simulink model "Allocation_Test"  (R2015a)
settings: Solver=ode45  StartTime=0.0  StopTime=10.0  RelTol=1e-3
undefined symbols (not defined in the file or in its folder): magnitude
libraries: aerolibutil x10, simulink_extras x6, simulink x2
settings Model: Creator=Nick  LastModifiedBy=Nick

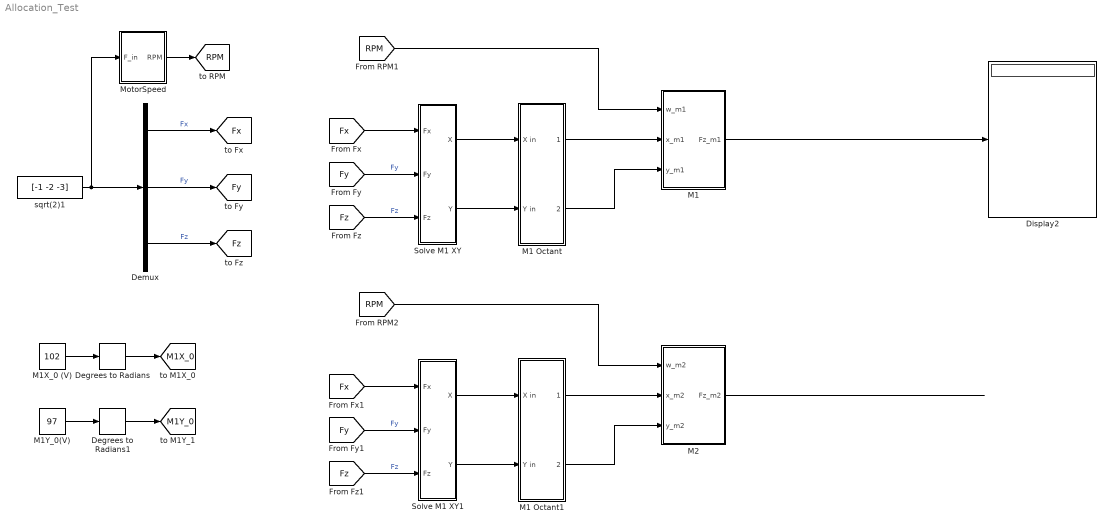
== system Allocation_Test ==
  Degrees to Radians : simulink_extras/Transformations/Degrees to Radians
  Degrees to Radians1 : simulink_extras/Transformations/Degrees to Radians
  Demux : Demux  Outputs=3
  Display2 : Display
      settings: Decimation=4
  M1 : Subsystem
  M1 Octant : Subsystem
  M1 Octant1 : Subsystem
  M1X_0 (V) : Constant  Value=102
  M1Y_0(V) : Constant  Value=97
  M2 : Subsystem
  MotorSpeed : Subsystem
  Solve M1 XY : Subsystem
  Solve M1 XY1 : Subsystem
  sqrt(2)1 : Constant  Value=[-1 -2 -3]
  tag scope: Fx=global, Fy=global, Fz=global, M1X_0=global, M1Y_0=global, RPM=global
  wires:
  sqrt(2)1/1 -> Demux/1, MotorSpeed/1(F_in)
  Demux/1 -> [Fx]  "Fx"
  Demux/2 -> [Fy]  "Fy"
  Demux/3 -> [Fz]  "Fz"
  MotorSpeed/1(RPM) -> [RPM]
  [Fz] -> Solve M1 XY/3(Fz)  "Fz"
  [Fx] -> Solve M1 XY/1(Fx)
  [Fy] -> Solve M1 XY/2(Fy)  "Fy"
  Solve M1 XY/2(Y) -> M1 Octant/2(Y in)
  Solve M1 XY/1(X) -> M1 Octant/1(X in)
  M1X_0 (V)/1 -> Degrees to Radians/1
  Degrees to Radians/1 -> [M1X_0]
  M1Y_0(V)/1 -> Degrees to Radians1/1
  Degrees to Radians1/1 -> [M1Y_0]
  [RPM] -> M1/1(w_m1)
  M1 Octant/2(Y Out) -> M1/3(y_m1)
  M1 Octant/1(X Out) -> M1/2(x_m1)
  M1/1(Fz_m1) -> Display2/1
  [Fz] -> Solve M1 XY1/3(Fz)  "Fz"
  [Fx] -> Solve M1 XY1/1(Fx)
  [Fy] -> Solve M1 XY1/2(Fy)  "Fy"
  Solve M1 XY1/2(Y) -> M1 Octant1/2(Y in)
  Solve M1 XY1/1(X) -> M1 Octant1/1(X in)
  [RPM] -> M2/1(w_m2)
  M1 Octant1/2(Y Out) -> M2/3(y_m2)
  M1 Octant1/1(X Out) -> M2/2(x_m2)
  M2/1(Fz_m2) -> ?

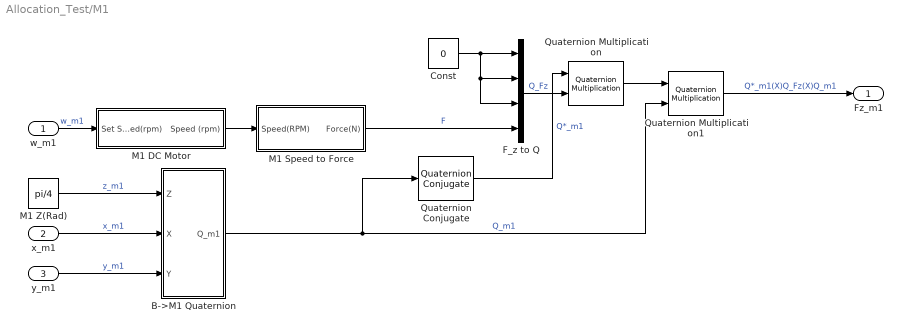
== system Allocation_Test/M1 ==
  w_m1 : Inport
  x_m1 : Inport  Port=2
  y_m1 : Inport  Port=3
  B->M1 Quaternion : Subsystem
  Const : Constant  Value=0
  F_z to Q : Concatenate  NumInputs=4
  M1 DC Motor : Subsystem
  M1 Speed to Force : Subsystem
  M1 Z(Rad) : Constant  Value=pi/4
  Quaternion Conjugate : aerolibutil/Quaternion Conjugate
  Quaternion Multiplication : aerolibutil/Quaternion Multiplication
  Quaternion Multiplication1 : aerolibutil/Quaternion Multiplication
  Fz_m1 : Outport
  wires:
  Quaternion Multiplication/1 -> Quaternion Multiplication1/1
  Const/1 -> F_z to Q/1, F_z to Q/3, F_z to Q/2
  M1 DC Motor/1(Speed (rpm)) -> M1 Speed to Force/1(Speed(RPM))
  B->M1 Quaternion/1(Q_m1) -> Quaternion Multiplication1/2, Quaternion Conjugate/1  "Q_m1"
  w_m1/1 -> M1 DC Motor/1(Set Speed(rpm))  "w_m1"
  F_z to Q/1 -> Quaternion Multiplication/2  "Q_Fz"
  M1 Z(Rad)/1 -> B->M1 Quaternion/1("Z ")  "z_m1"
  M1 Speed to Force/1(Force(N)) -> F_z to Q/4  "F"
  y_m1/1 -> B->M1 Quaternion/3(Y)  "y_m1"
  Quaternion Multiplication1/1 -> Fz_m1/1  "Q*_m1(X)Q_Fz(X)Q_m1"
  x_m1/1 -> B->M1 Quaternion/2(X)  "x_m1"
  Quaternion Conjugate/1 -> Quaternion Multiplication/1  "Q*_m1"

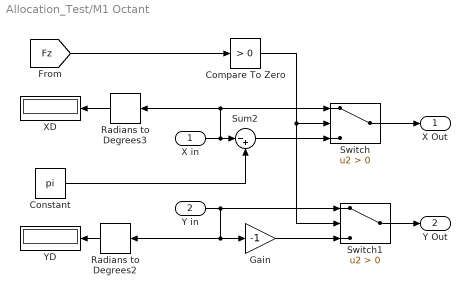
== system Allocation_Test/M1 Octant ==
  X in : Inport
  Y in : Inport  Port=2
  Compare To Zero : simulink/Logic and Bit Operations/Compare To Zero  relop=>  OutDataTypeStr=boolean
  Constant : Constant  Value=pi
  Gain : Gain  Gain=-1
  Radians to Degrees2 : simulink_extras/Transformations/Radians to Degrees
  Radians to Degrees3 : simulink_extras/Transformations/Radians to Degrees
  Sum2 : Sum  Inputs=|-+
  Switch : Switch  Criteria=u2 > Threshold
  Switch1 : Switch  Criteria=u2 > Threshold
  XD : Display
  YD : Display
  X Out : Outport
  Y Out : Outport  Port=2
  wires:
  Radians to Degrees2/1 -> YD/1
  Radians to Degrees3/1 -> XD/1
  Switch1/1 -> Y Out/1
  Sum2/1 -> Switch/3
  X in/1 -> Sum2/1, Switch/1, Radians to Degrees3/1
  Y in/1 -> Radians to Degrees2/1, Gain/1, Switch1/1
  Constant/1 -> Sum2/2
  Switch/1 -> X Out/1
  Gain/1 -> Switch1/3
  Compare To Zero/1 -> Switch1/2, Switch/2
  [Fz] -> Compare To Zero/1

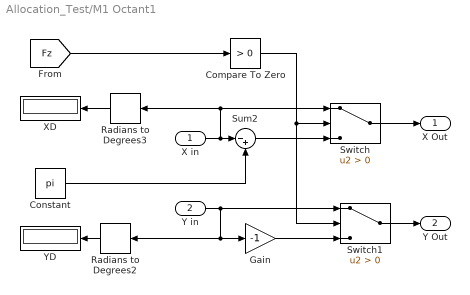
== system Allocation_Test/M1 Octant1 ==
  X in : Inport
  Y in : Inport  Port=2
  Compare To Zero : simulink/Logic and Bit Operations/Compare To Zero  relop=>  OutDataTypeStr=boolean
  Constant : Constant  Value=pi
  Gain : Gain  Gain=-1
  Radians to Degrees2 : simulink_extras/Transformations/Radians to Degrees
  Radians to Degrees3 : simulink_extras/Transformations/Radians to Degrees
  Sum2 : Sum  Inputs=|-+
  Switch : Switch  Criteria=u2 > Threshold
  Switch1 : Switch  Criteria=u2 > Threshold
  XD : Display
  YD : Display
  X Out : Outport
  Y Out : Outport  Port=2
  wires:
  Radians to Degrees2/1 -> YD/1
  Radians to Degrees3/1 -> XD/1
  Switch1/1 -> Y Out/1
  Sum2/1 -> Switch/3
  X in/1 -> Sum2/1, Switch/1, Radians to Degrees3/1
  Y in/1 -> Radians to Degrees2/1, Gain/1, Switch1/1
  Constant/1 -> Sum2/2
  Switch/1 -> X Out/1
  Gain/1 -> Switch1/3
  Compare To Zero/1 -> Switch1/2, Switch/2
  [Fz] -> Compare To Zero/1

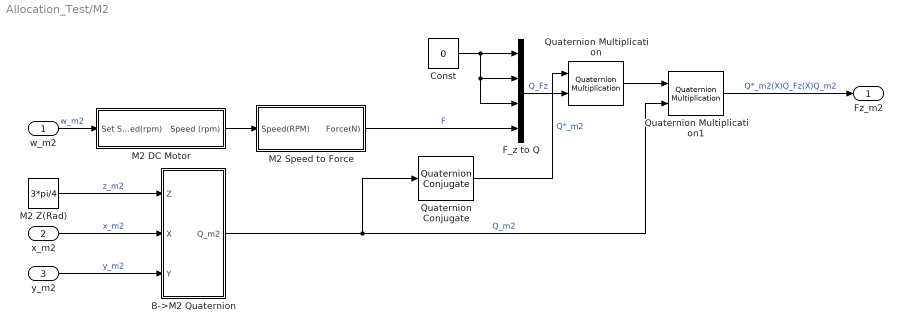
== system Allocation_Test/M2 ==
  w_m2 : Inport
  x_m2 : Inport  Port=2
  y_m2 : Inport  Port=3
  B->M2 Quaternion : Subsystem
  Const : Constant  Value=0
  F_z to Q : Concatenate  NumInputs=4
  M2 DC Motor : Subsystem
  M2 Speed to Force : Subsystem
  M2 Z(Rad) : Constant  Value=3*pi/4
  Quaternion Conjugate : aerolibutil/Quaternion Conjugate
  Quaternion Multiplication : aerolibutil/Quaternion Multiplication
  Quaternion Multiplication1 : aerolibutil/Quaternion Multiplication
  Fz_m2 : Outport
  wires:
  Quaternion Multiplication/1 -> Quaternion Multiplication1/1
  Const/1 -> F_z to Q/1, F_z to Q/3, F_z to Q/2
  M2 DC Motor/1(Speed (rpm)) -> M2 Speed to Force/1(Speed(RPM))
  B->M2 Quaternion/1(Q_m2) -> Quaternion Multiplication1/2, Quaternion Conjugate/1  "Q_m2"
  w_m2/1 -> M2 DC Motor/1(Set Speed(rpm))  "w_m2"
  F_z to Q/1 -> Quaternion Multiplication/2  "Q_Fz"
  M2 Z(Rad)/1 -> B->M2 Quaternion/1("Z ")  "z_m2"
  M2 Speed to Force/1(Force(N)) -> F_z to Q/4  "F"
  y_m2/1 -> B->M2 Quaternion/3(Y)  "y_m2"
  Quaternion Multiplication1/1 -> Fz_m2/1  "Q*_m2(X)Q_Fz(X)Q_m2"
  x_m2/1 -> B->M2 Quaternion/2(X)  "x_m2"
  Quaternion Conjugate/1 -> Quaternion Multiplication/1  "Q*_m2"

== system Allocation_Test/MotorSpeed ==
  F_in : Inport
  Divide : Product  Inputs=*/
  Force Coefficient CT : Constant  Value=0.000243
  Mins : Constant  Value=60
  Product : Product
  w^2 : Sqrt  SaturateOnIntegerOverflow=on
  |F| : Sqrt  SaturateOnIntegerOverflow=on
  |F|^2 : DotProduct  InputSameDT=on  OutDataTypeStr=Inherit: Inherit via internal rule
  RPM : Outport
  wires:
  w^2/1 -> Product/2
  Product/1 -> RPM/1  "RPM"
  Mins/1 -> Product/1
  Divide/1 -> w^2/1
  Force Coefficient CT/1 -> Divide/2
  F_in/1 -> |F|^2/2, |F|^2/1
  |F|^2/1 -> |F|/1
  |F|/1 -> Divide/1

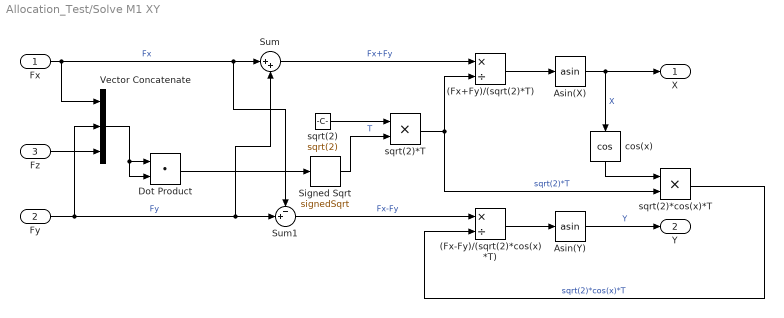
== system Allocation_Test/Solve M1 XY ==
  Fx : Inport
  Fy : Inport  Port=2
  Fz : Inport  Port=3
  (Fx+Fy)/(sqrt(2)*T) : Product  Inputs=*/
  (Fx-Fy)/(sqrt(2)*cos(x)*T) : Product  Inputs=*/
  Asin(X) : Trigonometry  Operator=asin
  Asin(Y) : Trigonometry  Operator=asin
  Dot Product : DotProduct  InputSameDT=on  OutDataTypeStr=Inherit: Inherit via internal rule
  Signed Sqrt : Sqrt  Operator=signedSqrt  SaturateOnIntegerOverflow=on
  Sum : Sum  Inputs=|++
  Sum1 : Sum  Inputs=-+|
  Vector Concatenate : Concatenate  NumInputs=3
  cos(x) : Trigonometry  Operator=cos
  sqrt(2) : Constant  Value=sqrt(2)
  sqrt(2)*T : Product
  sqrt(2)*cos(x)*T : Product
  X : Outport
  Y : Outport  Port=2
  wires:
  Fy/1 -> Vector Concatenate/2, Sum/2, Sum1/2  "Fy"
  Sum/1 -> (Fx+Fy)/(sqrt(2)*T)/1  "Fx+Fy"
  sqrt(2)/1 -> sqrt(2)*T/1
  cos(x)/1 -> sqrt(2)*cos(x)*T/1
  sqrt(2)*T/1 -> (Fx+Fy)/(sqrt(2)*T)/2, sqrt(2)*cos(x)*T/2  "sqrt(2)*T"
  (Fx+Fy)/(sqrt(2)*T)/1 -> Asin(X)/1
  sqrt(2)*cos(x)*T/1 -> (Fx-Fy)/(sqrt(2)*cos(x)*T)/2  "sqrt(2)*cos(x)*T"
  (Fx-Fy)/(sqrt(2)*cos(x)*T)/1 -> Asin(Y)/1
  Sum1/1 -> (Fx-Fy)/(sqrt(2)*cos(x)*T)/1  "Fx-Fy"
  Asin(Y)/1 -> Y/1  "Y"
  Asin(X)/1 -> X/1, cos(x)/1  "X"
  Fz/1 -> Vector Concatenate/3
  Signed Sqrt/1 -> sqrt(2)*T/2  "T"
  Fx/1 -> Sum1/1, Sum/1, Vector Concatenate/1  "Fx"
  Vector Concatenate/1 -> Dot Product/2, Dot Product/1
  Dot Product/1 -> Signed Sqrt/1

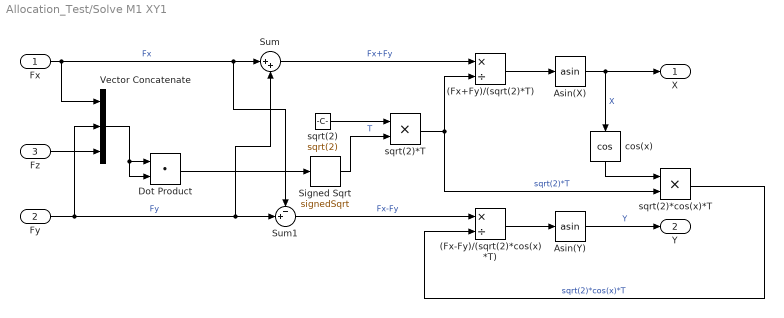
== system Allocation_Test/Solve M1 XY1 ==
  Fx : Inport
  Fy : Inport  Port=2
  Fz : Inport  Port=3
  (Fx+Fy)/(sqrt(2)*T) : Product  Inputs=*/
  (Fx-Fy)/(sqrt(2)*cos(x)*T) : Product  Inputs=*/
  Asin(X) : Trigonometry  Operator=asin
  Asin(Y) : Trigonometry  Operator=asin
  Dot Product : DotProduct  InputSameDT=on  OutDataTypeStr=Inherit: Inherit via internal rule
  Signed Sqrt : Sqrt  Operator=signedSqrt  SaturateOnIntegerOverflow=on
  Sum : Sum  Inputs=|++
  Sum1 : Sum  Inputs=-+|
  Vector Concatenate : Concatenate  NumInputs=3
  cos(x) : Trigonometry  Operator=cos
  sqrt(2) : Constant  Value=sqrt(2)
  sqrt(2)*T : Product
  sqrt(2)*cos(x)*T : Product
  X : Outport
  Y : Outport  Port=2
  wires:
  Fy/1 -> Vector Concatenate/2, Sum/2, Sum1/2  "Fy"
  Sum/1 -> (Fx+Fy)/(sqrt(2)*T)/1  "Fx+Fy"
  sqrt(2)/1 -> sqrt(2)*T/1
  cos(x)/1 -> sqrt(2)*cos(x)*T/1
  sqrt(2)*T/1 -> (Fx+Fy)/(sqrt(2)*T)/2, sqrt(2)*cos(x)*T/2  "sqrt(2)*T"
  (Fx+Fy)/(sqrt(2)*T)/1 -> Asin(X)/1
  sqrt(2)*cos(x)*T/1 -> (Fx-Fy)/(sqrt(2)*cos(x)*T)/2  "sqrt(2)*cos(x)*T"
  (Fx-Fy)/(sqrt(2)*cos(x)*T)/1 -> Asin(Y)/1
  Sum1/1 -> (Fx-Fy)/(sqrt(2)*cos(x)*T)/1  "Fx-Fy"
  Asin(Y)/1 -> Y/1  "Y"
  Asin(X)/1 -> X/1, cos(x)/1  "X"
  Fz/1 -> Vector Concatenate/3
  Signed Sqrt/1 -> sqrt(2)*T/2  "T"
  Fx/1 -> Sum1/1, Sum/1, Vector Concatenate/1  "Fx"
  Vector Concatenate/1 -> Dot Product/2, Dot Product/1
  Dot Product/1 -> Signed Sqrt/1

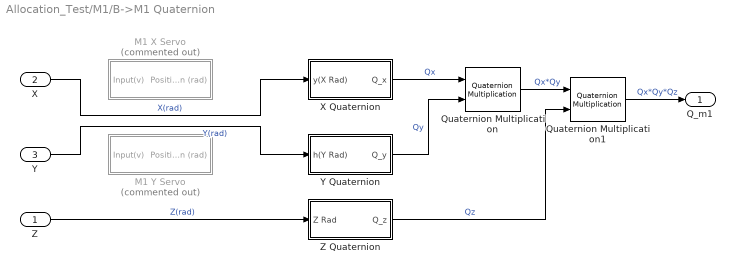
== system Allocation_Test/M1/B->M1 Quaternion ==
  "Z " : Inport
  X : Inport  Port=2
  Y : Inport  Port=3
  "M1 X Servo " : Subsystem  Commented=on
  M1 Y Servo : Subsystem  Commented=on
  Quaternion Multiplication : aerolibutil/Quaternion Multiplication
  Quaternion Multiplication1 : aerolibutil/Quaternion Multiplication
  X Quaternion : Subsystem
  Y Quaternion : Subsystem
  Z Quaternion : Subsystem
  Q_m1 : Outport
  wires:
  X/1 -> X Quaternion/1(y(X Rad))  "X(rad)"
  "Z "/1 -> Z Quaternion/1(Z Rad)  "Z(rad)"
  Quaternion Multiplication/1 -> Quaternion Multiplication1/1  "Qx*Qy"
  Quaternion Multiplication1/1 -> Q_m1/1  "Qx*Qy*Qz"
  Y/1 -> Y Quaternion/1(h(Y Rad))  "Y(rad)"
  X Quaternion/1(Q_x) -> Quaternion Multiplication/1  "Qx"
  Y Quaternion/1(Q_y) -> Quaternion Multiplication/2  "Qy"
  Z Quaternion/1(Q_z) -> Quaternion Multiplication1/2  "Qz"

== system Allocation_Test/M1/M1 DC Motor ==
  note: M1 DC Motor response
  Set Speed(rpm) : Inport
  ->ms : Product  Inputs=*/
  10080 Max : Saturate  UpperLimit=10080  LowerLimit=-10080
  Add : Sum
  Dead Time (ms) : Constant
  Dead Time Block : VariableTransportDelay  MaximumDelay=10
  Miliseconds : Constant  Value=1000
  Starting Speed : Constant  Value=10080
  Subtract : Sum  Inputs=+-
  Transfer Fcn : TransferFcn  Numerator=1  Denominator=[0.6 1]
  Speed (rpm) : Outport
  wires:
  Dead Time Block/1 -> Transfer Fcn/1
  Miliseconds/1 -> ->ms/2
  Dead Time (ms)/1 -> ->ms/1
  ->ms/1 -> Dead Time Block/2
  Transfer Fcn/1 -> 10080 Max/1
  Set Speed(rpm)/1 -> Subtract/1
  10080 Max/1 -> Add/1
  Add/1 -> Speed (rpm)/1
  Starting Speed/1 -> Add/2, Subtract/2
  Subtract/1 -> Dead Time Block/1

== system Allocation_Test/M1/M1 Speed to Force ==
  note: RPS to Force
  Speed(RPM) : Inport
  ->RPS : Product  Inputs=*/
  Force Coefficient CT : Constant  Value=0.000243
  M1 w^2 : Math  Operator=magnitude^2  SaturateOnIntegerOverflow=on
  Mins : Constant  Value=60
  Product : Product
  Force(N) : Outport
  wires:
  M1 w^2/1 -> Product/2
  ->RPS/1 -> M1 w^2/1
  Speed(RPM)/1 -> ->RPS/1
  Force Coefficient CT/1 -> Product/1
  Mins/1 -> ->RPS/2
  Product/1 -> Force(N)/1

== system Allocation_Test/M2/B->M2 Quaternion ==
  "Z " : Inport
  X : Inport  Port=2
  Y : Inport  Port=3
  "M1 X Servo " : Subsystem  Commented=on
  M1 Y Servo : Subsystem  Commented=on
  Quaternion Multiplication : aerolibutil/Quaternion Multiplication
  Quaternion Multiplication1 : aerolibutil/Quaternion Multiplication
  X Quaternion : Subsystem
  Y Quaternion : Subsystem
  Z Quaternion : Subsystem
  Q_m2 : Outport
  wires:
  X/1 -> X Quaternion/1(y(X Rad))  "X(rad)"
  "Z "/1 -> Z Quaternion/1(Z Rad)  "Z(rad)"
  Quaternion Multiplication/1 -> Quaternion Multiplication1/1  "Qx*Qy"
  Quaternion Multiplication1/1 -> Q_m2/1  "Qx*Qy*Qz"
  Y/1 -> Y Quaternion/1(h(Y Rad))  "Y(rad)"
  X Quaternion/1(Q_x) -> Quaternion Multiplication/1  "Qx"
  Y Quaternion/1(Q_y) -> Quaternion Multiplication/2  "Qy"
  Z Quaternion/1(Q_z) -> Quaternion Multiplication1/2  "Qz"

== system Allocation_Test/M2/M2 DC Motor ==
  note: M1 DC Motor response
  Set Speed(rpm) : Inport
  ->ms : Product  Inputs=*/
  10080 Max : Saturate  UpperLimit=10080  LowerLimit=-10080
  Add : Sum
  Dead Time (ms) : Constant
  Dead Time Block : VariableTransportDelay  MaximumDelay=10
  Miliseconds : Constant  Value=1000
  Starting Speed : Constant  Value=10080
  Subtract : Sum  Inputs=+-
  Transfer Fcn : TransferFcn  Numerator=1  Denominator=[0.6 1]
  Speed (rpm) : Outport
  wires:
  Dead Time Block/1 -> Transfer Fcn/1
  Miliseconds/1 -> ->ms/2
  Dead Time (ms)/1 -> ->ms/1
  ->ms/1 -> Dead Time Block/2
  Transfer Fcn/1 -> 10080 Max/1
  Set Speed(rpm)/1 -> Subtract/1
  10080 Max/1 -> Add/1
  Add/1 -> Speed (rpm)/1
  Starting Speed/1 -> Add/2, Subtract/2
  Subtract/1 -> Dead Time Block/1

== system Allocation_Test/M2/M2 Speed to Force ==
  note: RPS to Force
  Speed(RPM) : Inport
  ->RPS : Product  Inputs=*/
  Force Coefficient CT : Constant  Value=0.000243
  M1 w^2 : Math  Operator=magnitude^2  SaturateOnIntegerOverflow=on
  Mins : Constant  Value=60
  Product : Product
  Force(N) : Outport
  wires:
  M1 w^2/1 -> Product/2
  ->RPS/1 -> M1 w^2/1
  Speed(RPM)/1 -> ->RPS/1
  Force Coefficient CT/1 -> Product/1
  Mins/1 -> ->RPS/2
  Product/1 -> Force(N)/1

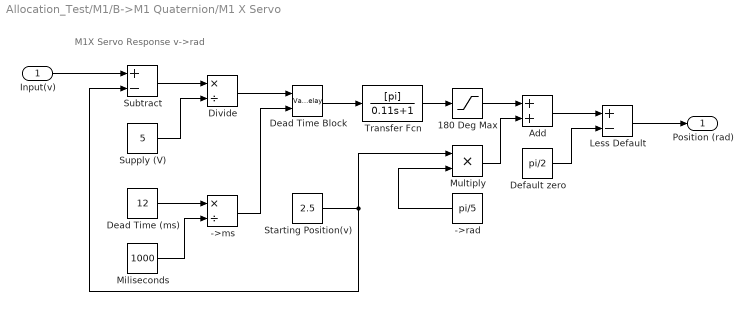
== system Allocation_Test/M1/B->M1 Quaternion/M1 X Servo  ==
  note: M1X Servo Response v->rad
  Input(v) : Inport
  ->ms : Product  Inputs=*/
  ->rad : Constant  Value=pi/5
  180 Deg Max : Saturate  UpperLimit=pi  LowerLimit=-pi
  Add : Sum
  Dead Time (ms) : Constant  Value=12
  Dead Time Block : VariableTransportDelay  MaximumDelay=10
  Default zero : Constant  Value=pi/2
  Divide : Product  Inputs=*/
  Less Default : Sum  Inputs=+-
  Miliseconds : Constant  Value=1000
  Multiply : Product  Inputs=**
  Starting Position(v) : Constant  Value=2.5
  Subtract : Sum  Inputs=+-
  Supply (V) : Constant  Value=5
  Transfer Fcn : TransferFcn  Numerator=[pi]  Denominator=[0.11 1]
  Position (rad) : Outport
  wires:
  Miliseconds/1 -> ->ms/2
  Dead Time (ms)/1 -> ->ms/1
  Default zero/1 -> Less Default/2
  Starting Position(v)/1 -> Multiply/1, Subtract/2
  Subtract/1 -> Divide/1
  Supply (V)/1 -> Divide/2
  Divide/1 -> Dead Time Block/1
  ->ms/1 -> Dead Time Block/2
  Dead Time Block/1 -> Transfer Fcn/1
  Transfer Fcn/1 -> 180 Deg Max/1
  180 Deg Max/1 -> Add/1
  ->rad/1 -> Multiply/2
  Multiply/1 -> Add/2
  Less Default/1 -> Position (rad)/1
  Add/1 -> Less Default/1
  Input(v)/1 -> Subtract/1

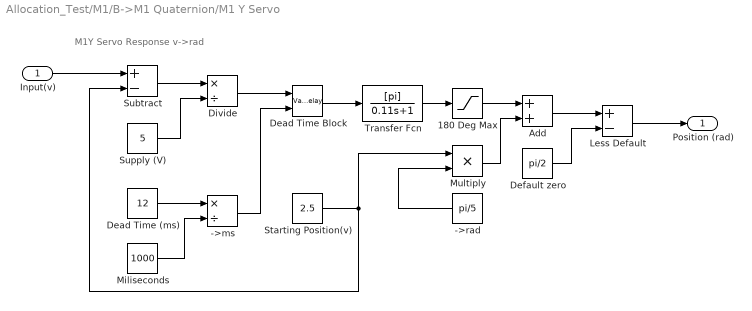
== system Allocation_Test/M1/B->M1 Quaternion/M1 Y Servo ==
  note: M1Y Servo Response v->rad
  Input(v) : Inport
  ->ms : Product  Inputs=*/
  ->rad : Constant  Value=pi/5
  180 Deg Max : Saturate  UpperLimit=pi  LowerLimit=-pi
  Add : Sum
  Dead Time (ms) : Constant  Value=12
  Dead Time Block : VariableTransportDelay  MaximumDelay=10
  Default zero : Constant  Value=pi/2
  Divide : Product  Inputs=*/
  Less Default : Sum  Inputs=+-
  Miliseconds : Constant  Value=1000
  Multiply : Product  Inputs=**
  Starting Position(v) : Constant  Value=2.5
  Subtract : Sum  Inputs=+-
  Supply (V) : Constant  Value=5
  Transfer Fcn : TransferFcn  Numerator=[pi]  Denominator=[0.11 1]
  Position (rad) : Outport
  wires:
  Miliseconds/1 -> ->ms/2
  Dead Time (ms)/1 -> ->ms/1
  Default zero/1 -> Less Default/2
  Starting Position(v)/1 -> Multiply/1, Subtract/2
  Subtract/1 -> Divide/1
  Supply (V)/1 -> Divide/2
  Divide/1 -> Dead Time Block/1
  ->ms/1 -> Dead Time Block/2
  Dead Time Block/1 -> Transfer Fcn/1
  Transfer Fcn/1 -> 180 Deg Max/1
  180 Deg Max/1 -> Add/1
  ->rad/1 -> Multiply/2
  Multiply/1 -> Add/2
  Less Default/1 -> Position (rad)/1
  Add/1 -> Less Default/1
  Input(v)/1 -> Subtract/1

== system Allocation_Test/M1/B->M1 Quaternion/X Quaternion ==
  y(X Rad) : Inport
  Const : Constant  Value=2
  Const1 : Constant  Value=0
  Divide : Product  Inputs=*/
  Trigonometric Function : Trigonometry  Operator=cos
  Trigonometric Function1 : Trigonometry
  Vector Concatenate : Concatenate  NumInputs=4
  Q_x : Outport
  wires:
  Vector Concatenate/1 -> Q_x/1
  Const/1 -> Divide/2
  Trigonometric Function1/1 -> Vector Concatenate/2
  Trigonometric Function/1 -> Vector Concatenate/1
  Const1/1 -> Vector Concatenate/4, Vector Concatenate/3
  Divide/1 -> Trigonometric Function1/1, Trigonometric Function/1
  y(X Rad)/1 -> Divide/1

== system Allocation_Test/M1/B->M1 Quaternion/Y Quaternion ==
  h(Y Rad) : Inport
  Const : Constant  Value=2
  Const1 : Constant  Value=0
  Divide : Product  Inputs=*/
  Trigonometric Function : Trigonometry  Operator=cos
  Trigonometric Function1 : Trigonometry
  Vector Concatenate : Concatenate  NumInputs=4
  Q_y : Outport
  wires:
  Vector Concatenate/1 -> Q_y/1
  Const/1 -> Divide/2
  Trigonometric Function/1 -> Vector Concatenate/1
  Const1/1 -> Vector Concatenate/2, Vector Concatenate/4
  Divide/1 -> Trigonometric Function1/1, Trigonometric Function/1
  h(Y Rad)/1 -> Divide/1
  Trigonometric Function1/1 -> Vector Concatenate/3

== system Allocation_Test/M1/B->M1 Quaternion/Z Quaternion ==
  Z Rad : Inport
  Const : Constant  Value=2
  Const1 : Constant  Value=0
  Divide : Product  Inputs=*/
  Trigonometric Function : Trigonometry  Operator=cos
  Trigonometric Function1 : Trigonometry
  Vector Concatenate : Concatenate  NumInputs=4
  Q_z : Outport
  wires:
  Vector Concatenate/1 -> Q_z/1
  Const/1 -> Divide/2
  Trigonometric Function/1 -> Vector Concatenate/1
  Const1/1 -> Vector Concatenate/3, Vector Concatenate/2
  Divide/1 -> Trigonometric Function1/1, Trigonometric Function/1
  Z Rad/1 -> Divide/1
  Trigonometric Function1/1 -> Vector Concatenate/4

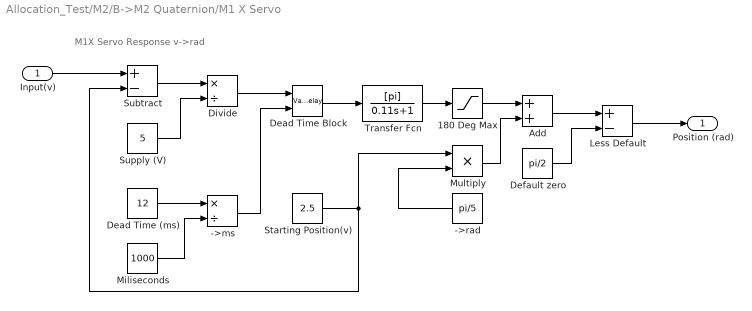
== system Allocation_Test/M2/B->M2 Quaternion/M1 X Servo  ==
  note: M1X Servo Response v->rad
  Input(v) : Inport
  ->ms : Product  Inputs=*/
  ->rad : Constant  Value=pi/5
  180 Deg Max : Saturate  UpperLimit=pi  LowerLimit=-pi
  Add : Sum
  Dead Time (ms) : Constant  Value=12
  Dead Time Block : VariableTransportDelay  MaximumDelay=10
  Default zero : Constant  Value=pi/2
  Divide : Product  Inputs=*/
  Less Default : Sum  Inputs=+-
  Miliseconds : Constant  Value=1000
  Multiply : Product  Inputs=**
  Starting Position(v) : Constant  Value=2.5
  Subtract : Sum  Inputs=+-
  Supply (V) : Constant  Value=5
  Transfer Fcn : TransferFcn  Numerator=[pi]  Denominator=[0.11 1]
  Position (rad) : Outport
  wires:
  Miliseconds/1 -> ->ms/2
  Dead Time (ms)/1 -> ->ms/1
  Default zero/1 -> Less Default/2
  Starting Position(v)/1 -> Multiply/1, Subtract/2
  Subtract/1 -> Divide/1
  Supply (V)/1 -> Divide/2
  Divide/1 -> Dead Time Block/1
  ->ms/1 -> Dead Time Block/2
  Dead Time Block/1 -> Transfer Fcn/1
  Transfer Fcn/1 -> 180 Deg Max/1
  180 Deg Max/1 -> Add/1
  ->rad/1 -> Multiply/2
  Multiply/1 -> Add/2
  Less Default/1 -> Position (rad)/1
  Add/1 -> Less Default/1
  Input(v)/1 -> Subtract/1

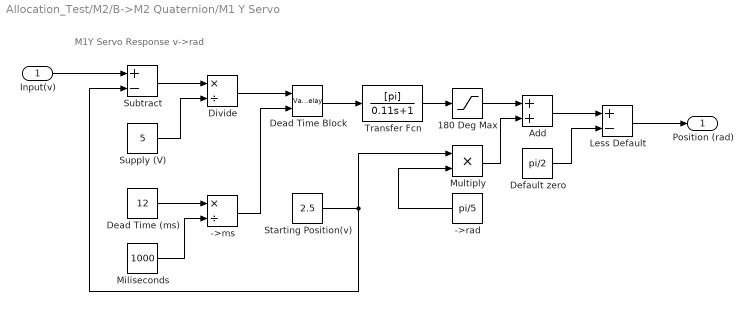
== system Allocation_Test/M2/B->M2 Quaternion/M1 Y Servo ==
  note: M1Y Servo Response v->rad
  Input(v) : Inport
  ->ms : Product  Inputs=*/
  ->rad : Constant  Value=pi/5
  180 Deg Max : Saturate  UpperLimit=pi  LowerLimit=-pi
  Add : Sum
  Dead Time (ms) : Constant  Value=12
  Dead Time Block : VariableTransportDelay  MaximumDelay=10
  Default zero : Constant  Value=pi/2
  Divide : Product  Inputs=*/
  Less Default : Sum  Inputs=+-
  Miliseconds : Constant  Value=1000
  Multiply : Product  Inputs=**
  Starting Position(v) : Constant  Value=2.5
  Subtract : Sum  Inputs=+-
  Supply (V) : Constant  Value=5
  Transfer Fcn : TransferFcn  Numerator=[pi]  Denominator=[0.11 1]
  Position (rad) : Outport
  wires:
  Miliseconds/1 -> ->ms/2
  Dead Time (ms)/1 -> ->ms/1
  Default zero/1 -> Less Default/2
  Starting Position(v)/1 -> Multiply/1, Subtract/2
  Subtract/1 -> Divide/1
  Supply (V)/1 -> Divide/2
  Divide/1 -> Dead Time Block/1
  ->ms/1 -> Dead Time Block/2
  Dead Time Block/1 -> Transfer Fcn/1
  Transfer Fcn/1 -> 180 Deg Max/1
  180 Deg Max/1 -> Add/1
  ->rad/1 -> Multiply/2
  Multiply/1 -> Add/2
  Less Default/1 -> Position (rad)/1
  Add/1 -> Less Default/1
  Input(v)/1 -> Subtract/1

== system Allocation_Test/M2/B->M2 Quaternion/X Quaternion ==
  y(X Rad) : Inport
  Const : Constant  Value=2
  Const1 : Constant  Value=0
  Divide : Product  Inputs=*/
  Trigonometric Function : Trigonometry  Operator=cos
  Trigonometric Function1 : Trigonometry
  Vector Concatenate : Concatenate  NumInputs=4
  Q_x : Outport
  wires:
  Vector Concatenate/1 -> Q_x/1
  Const/1 -> Divide/2
  Trigonometric Function1/1 -> Vector Concatenate/2
  Trigonometric Function/1 -> Vector Concatenate/1
  Const1/1 -> Vector Concatenate/4, Vector Concatenate/3
  Divide/1 -> Trigonometric Function1/1, Trigonometric Function/1
  y(X Rad)/1 -> Divide/1

== system Allocation_Test/M2/B->M2 Quaternion/Y Quaternion ==
  h(Y Rad) : Inport
  Const : Constant  Value=2
  Const1 : Constant  Value=0
  Divide : Product  Inputs=*/
  Trigonometric Function : Trigonometry  Operator=cos
  Trigonometric Function1 : Trigonometry
  Vector Concatenate : Concatenate  NumInputs=4
  Q_y : Outport
  wires:
  Vector Concatenate/1 -> Q_y/1
  Const/1 -> Divide/2
  Trigonometric Function/1 -> Vector Concatenate/1
  Const1/1 -> Vector Concatenate/2, Vector Concatenate/4
  Divide/1 -> Trigonometric Function1/1, Trigonometric Function/1
  h(Y Rad)/1 -> Divide/1
  Trigonometric Function1/1 -> Vector Concatenate/3

== system Allocation_Test/M2/B->M2 Quaternion/Z Quaternion ==
  Z Rad : Inport
  Const : Constant  Value=2
  Const1 : Constant  Value=0
  Divide : Product  Inputs=*/
  Trigonometric Function : Trigonometry  Operator=cos
  Trigonometric Function1 : Trigonometry
  Vector Concatenate : Concatenate  NumInputs=4
  Q_z : Outport
  wires:
  Vector Concatenate/1 -> Q_z/1
  Const/1 -> Divide/2
  Trigonometric Function/1 -> Vector Concatenate/1
  Const1/1 -> Vector Concatenate/3, Vector Concatenate/2
  Divide/1 -> Trigonometric Function1/1, Trigonometric Function/1
  Z Rad/1 -> Divide/1
  Trigonometric Function1/1 -> Vector Concatenate/4
